simulink model "AnomalyResponseDelay"  (R2017b)
settings: Solver=FixedStepAuto  StartTime=0.0  StopTime=tfin  FixedStep=dT  MinStep=1e-5  RelTol=1e-6
values from neighbouring files (symbols this model uses):
  gamma = 10    [AnomalyResponseSim.m]
  tau = SP.tau    [AnomalyResponseSim.m]    (also in thesis_plots.m)
  ts = SP.ts    [AnomalyResponseSim.m]    (also in thesis_plots.m)
  ts_rm = SP.ts_rm    [AnomalyResponseSim.m]    (also in thesis_plots.m)
undefined symbols (not defined in the file or in its folder): Am, Am_3d, Ap, Bm, Bm_3d, Bp, dT, gamma_3d_q, gamma_3d_th, Lm, Lm_3d, P, P_3d, q0, q_0, Theta_0, theta_0_1, theta_0_2
libraries: vrlib x14, simulink x4
settings Model: Creator=ben  LastModifiedBy=ben
settings SolverCC: ShapePreserveControl=EnableAll  ZeroCrossControl=EnableAll
settings DataIOCC: SaveOutput=off  SignalLogging=off  DSMLogging=off  ReturnWorkspaceOutputs=on  ReturnWorkspaceOutputsName=simout
settings CodeAppCC: StateflowObjectComments=on

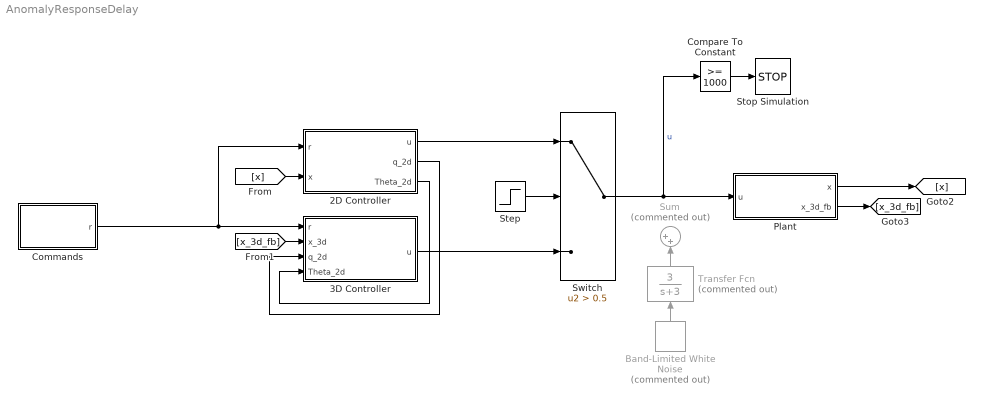
== system AnomalyResponseDelay ==
  2D Controller : Subsystem
  3D Controller : Subsystem
  Band-Limited White Noise : simulink/Sources/Band-Limited White Noise  Commented=on  Cov=[0.2]  Ts=0.05  seed=[23341]
  Commands : Subsystem
  Compare To Constant : simulink/Logic and Bit Operations/Compare To Constant  relop=>=  const=1000  OutDataTypeStr=boolean
  Plant : Subsystem
  Step : Step  Time=ts_rm  Before=1  After=0  SampleTime=0
  Stop Simulation : Stop
  Sum : Sum  Commented=on  Inputs=|++
  Switch : Switch  Criteria=u2 > Threshold  Threshold=0.5
  Transfer Fcn : TransferFcn  Commented=on  Numerator=[3]  Denominator=[1 3]
  wires:
  Plant/1(x) -> [x]
  Plant/2(x_3d_fb) -> [x_3d_fb]
  [x] -> 2D Controller/2(x)
  [x_3d_fb] -> 3D Controller/2(x_3d)
  Step/1 -> Switch/2
  Switch/1 -> Compare To Constant/1, Plant/1(u)  "u"
  3D Controller/1(u) -> Switch/3
  2D Controller/1(u) -> Switch/1
  2D Controller/3(Theta_2d) -> 3D Controller/4(Theta_2d)
  2D Controller/2(q_2d) -> 3D Controller/3(q_2d)
  Commands/1(r) -> 2D Controller/1(r), 3D Controller/1(r)
  Band-Limited White Noise/1 -> Transfer Fcn/1
  Transfer Fcn/1 -> Sum/2
  Compare To Constant/1 -> Stop Simulation/1

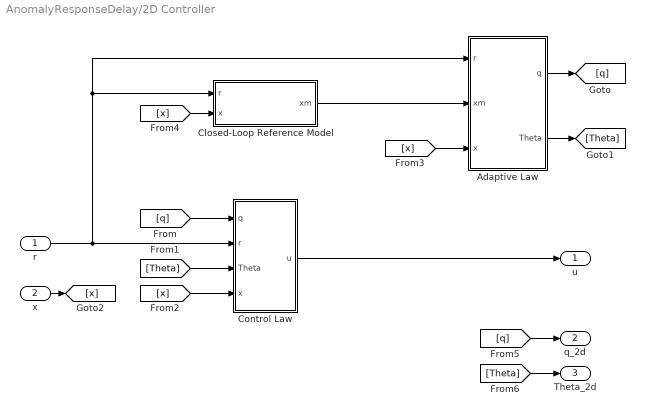
== system AnomalyResponseDelay/2D Controller ==
  r : Inport
  x : Inport  Port=2
  Adaptive Law : Subsystem
  Closed-Loop Reference Model : Subsystem
  Control Law : Subsystem
  u : Outport
  q_2d : Outport  Port=2
  Theta_2d : Outport  Port=3
  wires:
  Closed-Loop Reference Model/1(xm) -> Adaptive Law/2(xm)
  [x] -> Control Law/4(x)
  [q] -> Control Law/1(q)
  [Theta] -> Control Law/3(Theta)
  Adaptive Law/2(Theta) -> [Theta]
  r/1 -> Closed-Loop Reference Model/1(r), Adaptive Law/1(r), Control Law/2(r)
  [x] -> Closed-Loop Reference Model/2(x)
  [x] -> Adaptive Law/3(x)
  Adaptive Law/1(q) -> [q]
  Control Law/1(u) -> u/1
  x/1 -> [x]
  [q] -> q_2d/1
  [Theta] -> Theta_2d/1

== system AnomalyResponseDelay/3D Controller ==
  r : Inport
  x_3d : Inport  Port=2
  q_2d : Inport  Port=3
  Theta_2d : Inport  Port=4
  Adaptive Law : Subsystem
  Closed-Loop Reference Model : Subsystem
  Control Law : Subsystem
  u : Outport
  wires:
  Control Law/1(u) -> u/1
  Adaptive Law/1(q) -> [q_3d]
  [x_3d] -> Adaptive Law/3(x)
  [x_3d] -> Closed-Loop Reference Model/2(x)
  r/1 -> Control Law/2(r), Adaptive Law/1(r), Closed-Loop Reference Model/1(r)
  Adaptive Law/2(Theta) -> [Theta_3d]
  [Theta_3d] -> Control Law/3(Theta)
  [q_3d] -> Control Law/1(q)
  [x_3d] -> Control Law/4(x)
  Closed-Loop Reference Model/1(xm) -> Adaptive Law/2(xm)
  x_3d/1 -> [x_3d]
  Theta_2d/1 -> Adaptive Law/5(Theta_2d)
  q_2d/1 -> Adaptive Law/4(q_2d)

== system AnomalyResponseDelay/Commands ==
  From Workspace : FromWorkspace  VariableName=r_timed  SampleTime=0  Interpolate=off  OutputAfterFinalValue=Setting to zero
  To Workspace : ToWorkspace  VariableName=r  SampleTime=-1
      settings: Save2DSignal=2-D array (concatenate along first dimension)
  r : Outport
  wires:
  From Workspace/1 -> To Workspace/1, r/1

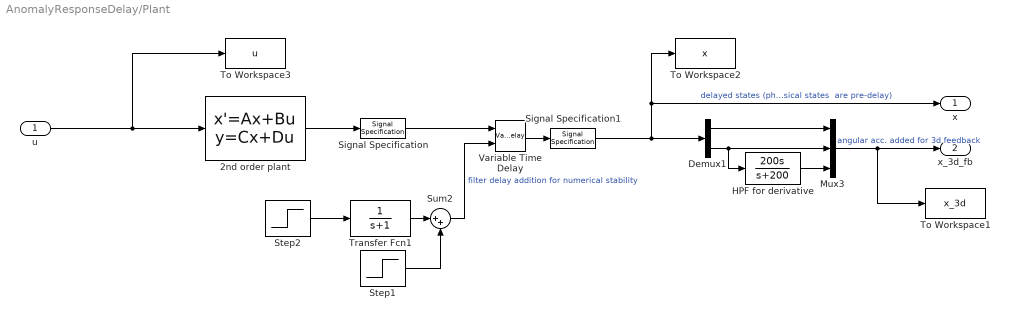
== system AnomalyResponseDelay/Plant ==
  u : Inport
  2nd order plant : StateSpace  A=Ap  B=Bp  C=eye(2)  D=[0; 0]  InitialCondition=0
  Demux1 : Demux  Outputs=[1 1]
  HPF for derivative : TransferFcn  Numerator=[200 0]  Denominator=[1 200]
  Mux3 : Mux  Inputs=[1 1 1]
  Signal Specification : SignalSpecification  Dimensions=[2 1]
  Signal Specification1 : SignalSpecification  Dimensions=[2 1]
  Step1 : Step  Time=ts  After=dT  SampleTime=0
  Step2 : Step  Time=ts  After=tau-dT  SampleTime=0
  Sum2 : Sum  Inputs=|++
  To Workspace1 : ToWorkspace  VariableName=x_3d  SampleTime=-1
      settings: Save2DSignal=2-D array (concatenate along first dimension)
  To Workspace2 : ToWorkspace  VariableName=x  SampleTime=-1
  To Workspace3 : ToWorkspace  VariableName=u  SampleTime=-1
      settings: Save2DSignal=2-D array (concatenate along first dimension)
  Transfer Fcn1 : TransferFcn  Denominator=[1 1]
  Variable Time Delay : VariableTransportDelay  MaximumDelay=tau*1.01  ZeroDelay=on
  x : Outport
  x_3d_fb : Outport  Port=2
  wires:
  Variable Time Delay/1 -> Signal Specification1/1
  Step2/1 -> Transfer Fcn1/1
  Sum2/1 -> Variable Time Delay/2  "filter delay addition for numerical stability"
  2nd order plant/1 -> Signal Specification/1
  u/1 -> 2nd order plant/1, To Workspace3/1
  Demux1/1 -> Mux3/1
  Demux1/2 -> HPF for derivative/1, Mux3/2
  HPF for derivative/1 -> Mux3/3
  Mux3/1 -> To Workspace1/1, x_3d_fb/1  "angular acc. added for 3d feedback"
  Signal Specification/1 -> Variable Time Delay/1
  Signal Specification1/1 -> Demux1/1, To Workspace2/1, x/1  "delayed states (physical states  are pre-delay)"
  Transfer Fcn1/1 -> Sum2/1
  Step1/1 -> Sum2/2

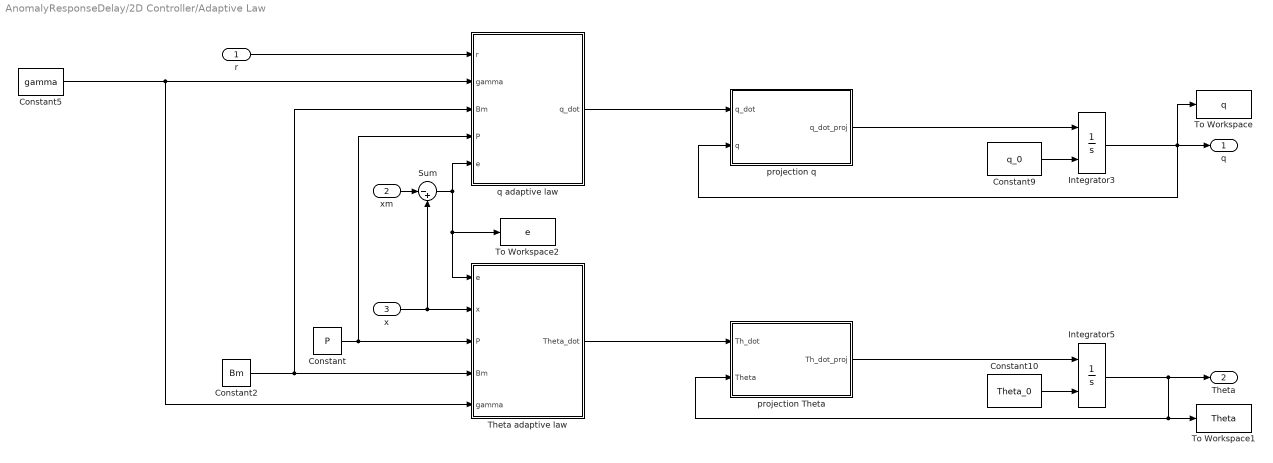
== system AnomalyResponseDelay/2D Controller/Adaptive Law ==
  r : Inport
  xm : Inport  Port=2  PortDimensions=[2,1]
  x : Inport  Port=3  PortDimensions=[2,1]
  Constant : Constant  Value=P  VectorParams1D=off
  Constant10 : Constant  Value=Theta_0  VectorParams1D=off
  Constant2 : Constant  Value=Bm  VectorParams1D=off
  Constant5 : Constant  Value=gamma  VectorParams1D=off
  Constant9 : Constant  Value=q_0  VectorParams1D=off
  Integrator3 : Integrator  InitialConditionSource=external  InitialCondition=q0
  Integrator5 : Integrator  InitialConditionSource=external
  Sum : Sum  Inputs=|-+
  Theta adaptive law : MATLAB Function  TreatAsAtomicUnit=on
  To Workspace : ToWorkspace  VariableName=q  SampleTime=-1
      settings: Save2DSignal=2-D array (concatenate along first dimension)
  To Workspace1 : ToWorkspace  VariableName=Theta  SampleTime=-1
      settings: Save2DSignal=2-D array (concatenate along first dimension)
  To Workspace2 : ToWorkspace  VariableName=e  SampleTime=-1
  projection Theta : Subsystem
  projection q : Subsystem
  q adaptive law : MATLAB Function  TreatAsAtomicUnit=on
  q : Outport
  Theta : Outport  Port=2
  wires:
  x/1 -> Theta adaptive law/2(x), Sum/2
  Constant/1 -> Theta adaptive law/3(P), q adaptive law/4(P)
  xm/1 -> Sum/1
  Sum/1 -> To Workspace2/1, Theta adaptive law/1(e), q adaptive law/5(e)
  Constant2/1 -> Theta adaptive law/4(Bm), q adaptive law/3(Bm)
  Constant5/1 -> Theta adaptive law/5(gamma), q adaptive law/2(gamma)
  r/1 -> q adaptive law/1(r)
  Constant9/1 -> Integrator3/2
  Integrator3/1 -> To Workspace/1, q/1, projection q/2(q)
  Constant10/1 -> Integrator5/2
  Integrator5/1 -> Theta/1, projection Theta/2(Theta), To Workspace1/1
  Theta adaptive law/1(Theta_dot) -> projection Theta/1(Th_dot)
  projection Theta/1(Th_dot_proj) -> Integrator5/1
  q adaptive law/1(q_dot) -> projection q/1(q_dot)
  projection q/1(q_dot_proj) -> Integrator3/1

== system AnomalyResponseDelay/2D Controller/Closed-Loop Reference Model ==
  r : Inport
  x : Inport  Port=2
  Am : Gain  Gain=Am  Multiplication=Matrix(K*u)
  Bm : Gain  Gain=Bm  Multiplication=Matrix(K*u)
  Integrator : Integrator
  Lm : Gain  Gain=Lm  Multiplication=Matrix(K*u)
  Sum2 : Sum  Inputs=-+|
  Sum3 : Sum  Inputs=-++
  To Workspace1 : ToWorkspace  VariableName=xm  SampleTime=-1
      settings: Save2DSignal=2-D array (concatenate along first dimension)
  xm : Outport
  wires:
  Integrator/1 -> Am/1, To Workspace1/1, xm/1, Sum2/1
  r/1 -> Bm/1
  x/1 -> Sum2/2
  Sum3/1 -> Integrator/1
  Bm/1 -> Sum3/2
  Lm/1 -> Sum3/1
  Sum2/1 -> Lm/1
  Am/1 -> Sum3/3

== system AnomalyResponseDelay/2D Controller/Control Law ==
  q : Inport
  r : Inport  Port=2
  Theta : Inport  Port=3
  x : Inport  Port=4
  Product : Product  Multiplication=Matrix(*)
  Sum : Sum  Inputs=|++
  q*r : Product
  u : Outport
  wires:
  x/1 -> Product/2
  q/1 -> q*r/1
  Product/1 -> Sum/2
  r/1 -> q*r/2
  q*r/1 -> Sum/1
  Sum/1 -> u/1
  Theta/1 -> Product/1

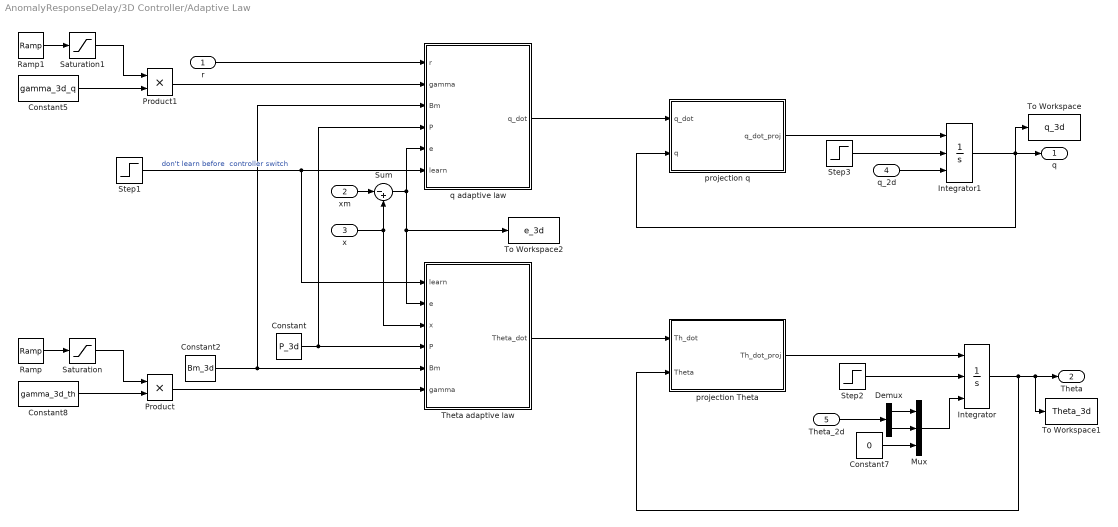
== system AnomalyResponseDelay/3D Controller/Adaptive Law ==
  r : Inport
  xm : Inport  Port=2  PortDimensions=[3,1]
  x : Inport  Port=3  PortDimensions=[3,1]
  q_2d : Inport  Port=4
  Theta_2d : Inport  Port=5
  Constant : Constant  Value=P_3d  VectorParams1D=off
  Constant2 : Constant  Value=Bm_3d  VectorParams1D=off
  Constant5 : Constant  Value=gamma_3d_q  VectorParams1D=off
  Constant7 : Constant  Value=0
  Constant8 : Constant  Value=gamma_3d_th  VectorParams1D=off
  Demux : Demux  Outputs=2
  Integrator : Integrator  ExternalReset=falling  InitialConditionSource=external
  Integrator1 : Integrator  ExternalReset=falling  InitialConditionSource=external  InitialCondition=q0
  Mux : Mux  Inputs=3
  Product : Product
  Product1 : Product
  Ramp : simulink/Sources/Ramp  slope=0.1  start=ts_rm  X0=0
  Ramp1 : simulink/Sources/Ramp  slope=0.1  start=ts_rm  X0=0
  Saturation : Saturate  UpperLimit=1  LowerLimit=0
  Saturation1 : Saturate  UpperLimit=1  LowerLimit=0
  Step1 : Step  Time=ts_rm  SampleTime=0
  Step2 : Step  Time=ts_rm  Before=0.5  After=-0.5  SampleTime=0
  Step3 : Step  Time=ts_rm  Before=0.5  After=-0.5  SampleTime=0
  Sum : Sum  Inputs=|-+
  Theta adaptive law : MATLAB Function  TreatAsAtomicUnit=on
  To Workspace : ToWorkspace  VariableName=q_3d  SampleTime=-1
      settings: Save2DSignal=2-D array (concatenate along first dimension)
  To Workspace1 : ToWorkspace  VariableName=Theta_3d  SampleTime=-1
      settings: Save2DSignal=2-D array (concatenate along first dimension)
  To Workspace2 : ToWorkspace  VariableName=e_3d  SampleTime=-1
  projection Theta : Subsystem
  projection q : Subsystem
  q adaptive law : MATLAB Function  TreatAsAtomicUnit=on
  q : Outport
  Theta : Outport  Port=2
  wires:
  r/1 -> q adaptive law/1(r)
  Constant2/1 -> q adaptive law/3(Bm), Theta adaptive law/5(Bm)
  Sum/1 -> q adaptive law/5(e), To Workspace2/1, Theta adaptive law/2(e)
  xm/1 -> Sum/1
  Constant/1 -> q adaptive law/4(P), Theta adaptive law/4(P)
  x/1 -> Theta adaptive law/3(x), Sum/2
  Step2/1 -> Integrator/2
  Step3/1 -> Integrator1/2
  Demux/1 -> Mux/1
  Demux/2 -> Mux/2
  Theta_2d/1 -> Demux/1
  Constant7/1 -> Mux/3
  Mux/1 -> Integrator/3
  Integrator1/1 -> projection q/2(q), q/1, To Workspace/1
  Integrator/1 -> projection Theta/2(Theta), Theta/1, To Workspace1/1
  q adaptive law/1(q_dot) -> projection q/1(q_dot)
  projection q/1(q_dot_proj) -> Integrator1/1
  Theta adaptive law/1(Theta_dot) -> projection Theta/1(Th_dot)
  projection Theta/1(Th_dot_proj) -> Integrator/1
  q_2d/1 -> Integrator1/3
  Product1/1 -> q adaptive law/2(gamma)
  Product/1 -> Theta adaptive law/6(gamma)
  Constant8/1 -> Product/2
  Ramp/1 -> Saturation/1
  Step1/1 -> Theta adaptive law/1(learn), q adaptive law/6(learn)  "don't learn before  controller switch"
  Saturation/1 -> Product/1
  Constant5/1 -> Product1/2
  Ramp1/1 -> Saturation1/1
  Saturation1/1 -> Product1/1

== system AnomalyResponseDelay/3D Controller/Closed-Loop Reference Model ==
  r : Inport
  x : Inport  Port=2
  Am : Gain  Gain=Am_3d  Multiplication=Matrix(K*u)
  Bm : Gain  Gain=Bm_3d  Multiplication=Matrix(K*u)
  Integrator : Integrator
  Lm : Gain  Gain=Lm_3d  Multiplication=Matrix(K*u)
  Sum2 : Sum  Inputs=-+|
  Sum3 : Sum  Inputs=-++
  To Workspace1 : ToWorkspace  VariableName=xm_3d  SampleTime=-1
      settings: Save2DSignal=2-D array (concatenate along first dimension)
  xm : Outport
  wires:
  Am/1 -> Sum3/3
  Sum2/1 -> Lm/1
  Lm/1 -> Sum3/1
  Bm/1 -> Sum3/2
  x/1 -> Sum2/2
  r/1 -> Bm/1
  Integrator/1 -> Sum2/1, xm/1, To Workspace1/1, Am/1
  Sum3/1 -> Integrator/1

== system AnomalyResponseDelay/3D Controller/Control Law ==
  q : Inport
  r : Inport  Port=2
  Theta : Inport  Port=3
  x : Inport  Port=4
  Product : Product  Multiplication=Matrix(*)
  Sum : Sum  Inputs=|++
  q*r : Product
  u : Outport
  wires:
  x/1 -> Product/2
  q/1 -> q*r/1
  Product/1 -> Sum/2
  r/1 -> q*r/2
  q*r/1 -> Sum/1
  Sum/1 -> u/1
  Theta/1 -> Product/1

== system AnomalyResponseDelay/2D Controller/Adaptive Law/projection Theta ==
  Th_dot : Inport
  Theta : Inport  Port=2
  Demux : Demux  Outputs=2
  Demux1 : Demux  Outputs=2
  Math Function : Math  Operator=transpose  SaturateOnIntegerOverflow=on
  Mux : Mux  Inputs=2
  Projection Block : Subsystem  mask{Epsilon=50, thetamax=200, Prcenter=0, Pr0=theta_0_1}
      mask prompts: thetamax "Bound (radius of the ball)"; Prcenter "Center of the Ball"; Pr0 "Initialization of integral"
      mask help:
      | Computes projection of the signal and safely integrate it.
      | Works both for scalar and vector signals.
      | It considers the parameter set as a ball at the specified location with
      | preset radius.
      mask init:
      | innerradius=thetamax/sqrt(1+Epsilon);
      | Intmax=thetamax+Prcenter;
      | Intmin=-thetamax+Prcenter;
      | Thetamax=innerradius;
  Projection Block1 : Subsystem  mask{Epsilon=100, thetamax=50, Prcenter=0, Pr0=theta_0_2}
      mask prompts: thetamax "Bound (radius of the ball)"; Prcenter "Center of the Ball"; Pr0 "Initialization of integral"
      mask help:
      | Computes projection of the signal and safely integrate it.
      | Works both for scalar and vector signals.
      | It considers the parameter set as a ball at the specified location with
      | preset radius.
      mask init:
      | innerradius=thetamax/sqrt(1+Epsilon);
      | Intmax=thetamax+Prcenter;
      | Intmin=-thetamax+Prcenter;
      | Thetamax=innerradius;
  Th_dot_proj : Outport
  wires:
  Math Function/1 -> Th_dot_proj/1
  Projection Block/1(proj) -> Mux/1
  Demux/1 -> Projection Block/2(y)
  Projection Block1/1(proj) -> Mux/2
  Demux/2 -> Projection Block1/2(y)
  Th_dot/1 -> Demux/1
  Mux/1 -> Math Function/1
  Theta/1 -> Demux1/1
  Demux1/1 -> Projection Block/1(theta)
  Demux1/2 -> Projection Block1/1(theta)

== system AnomalyResponseDelay/2D Controller/Adaptive Law/projection q ==
  q_dot : Inport
  q : Inport  Port=2
  Projection Block : Subsystem  mask{Epsilon=50, thetamax=200, Prcenter=0, Pr0=q_0}
      mask prompts: thetamax "Bound (radius of the ball)"; Prcenter "Center of the Ball"; Pr0 "Initialization of integral"
      mask help:
      | Computes projection of the signal and safely integrate it.
      | Works both for scalar and vector signals.
      | It considers the parameter set as a ball at the specified location with
      | preset radius.
      mask init:
      | innerradius=thetamax/sqrt(1+Epsilon);
      | Intmax=thetamax+Prcenter;
      | Intmin=-thetamax+Prcenter;
      | Thetamax=innerradius;
  q_dot_proj : Outport
  wires:
  q_dot/1 -> Projection Block/2(y)
  Projection Block/1(proj) -> q_dot_proj/1
  q/1 -> Projection Block/1(theta)

== system AnomalyResponseDelay/3D Controller/Adaptive Law/projection Theta ==
  Th_dot : Inport
  Theta : Inport  Port=2
  Demux : Demux  Outputs=3
  Demux1 : Demux  Outputs=3
  Math Function : Math  Operator=transpose  SaturateOnIntegerOverflow=on
  Mux : Mux  Inputs=3
  Projection Block : Subsystem  mask{Epsilon=50, thetamax=200, Prcenter=0, Pr0=theta_0_1}
      mask prompts: thetamax "Bound (radius of the ball)"; Prcenter "Center of the Ball"; Pr0 "Initialization of integral"
      mask help:
      | Computes projection of the signal and safely integrate it.
      | Works both for scalar and vector signals.
      | It considers the parameter set as a ball at the specified location with
      | preset radius.
      mask init:
      | innerradius=thetamax/sqrt(1+Epsilon);
      | Intmax=thetamax+Prcenter;
      | Intmin=-thetamax+Prcenter;
      | Thetamax=innerradius;
  Projection Block1 : Subsystem  mask{Epsilon=50, thetamax=75, Prcenter=0, Pr0=theta_0_2}
      mask prompts: thetamax "Bound (radius of the ball)"; Prcenter "Center of the Ball"; Pr0 "Initialization of integral"
      mask help:
      | Computes projection of the signal and safely integrate it.
      | Works both for scalar and vector signals.
      | It considers the parameter set as a ball at the specified location with
      | preset radius.
      mask init:
      | innerradius=thetamax/sqrt(1+Epsilon);
      | Intmax=thetamax+Prcenter;
      | Intmin=-thetamax+Prcenter;
      | Thetamax=innerradius;
  Projection Block2 : Subsystem  mask{Epsilon=5, thetamax=10, Prcenter=0, Pr0=0}
      mask prompts: thetamax "Bound (radius of the ball)"; Prcenter "Center of the Ball"; Pr0 "Initialization of integral"
      mask help:
      | Computes projection of the signal and safely integrate it.
      | Works both for scalar and vector signals.
      | It considers the parameter set as a ball at the specified location with
      | preset radius.
      mask init:
      | innerradius=thetamax/sqrt(1+Epsilon);
      | Intmax=thetamax+Prcenter;
      | Intmin=-thetamax+Prcenter;
      | Thetamax=innerradius;
  Th_dot_proj : Outport
  wires:
  Math Function/1 -> Th_dot_proj/1
  Projection Block/1(proj) -> Mux/1
  Demux/1 -> Projection Block/2(y)
  Projection Block1/1(proj) -> Mux/2
  Demux/2 -> Projection Block1/2(y)
  Th_dot/1 -> Demux/1
  Mux/1 -> Math Function/1
  Theta/1 -> Demux1/1
  Demux1/1 -> Projection Block/1(theta)
  Demux1/2 -> Projection Block1/1(theta)
  Projection Block2/1(proj) -> Mux/3
  Demux/3 -> Projection Block2/2(y)
  Demux1/3 -> Projection Block2/1(theta)

== system AnomalyResponseDelay/3D Controller/Adaptive Law/projection q ==
  q_dot : Inport
  q : Inport  Port=2
  Projection Block : Subsystem  mask{Epsilon=50, thetamax=200, Prcenter=0, Pr0=q_0}
      mask prompts: thetamax "Bound (radius of the ball)"; Prcenter "Center of the Ball"; Pr0 "Initialization of integral"
      mask help:
      | Computes projection of the signal and safely integrate it.
      | Works both for scalar and vector signals.
      | It considers the parameter set as a ball at the specified location with
      | preset radius.
      mask init:
      | innerradius=thetamax/sqrt(1+Epsilon);
      | Intmax=thetamax+Prcenter;
      | Intmin=-thetamax+Prcenter;
      | Thetamax=innerradius;
  q_dot_proj : Outport
  wires:
  q_dot/1 -> Projection Block/2(y)
  Projection Block/1(proj) -> q_dot_proj/1
  q/1 -> Projection Block/1(theta)

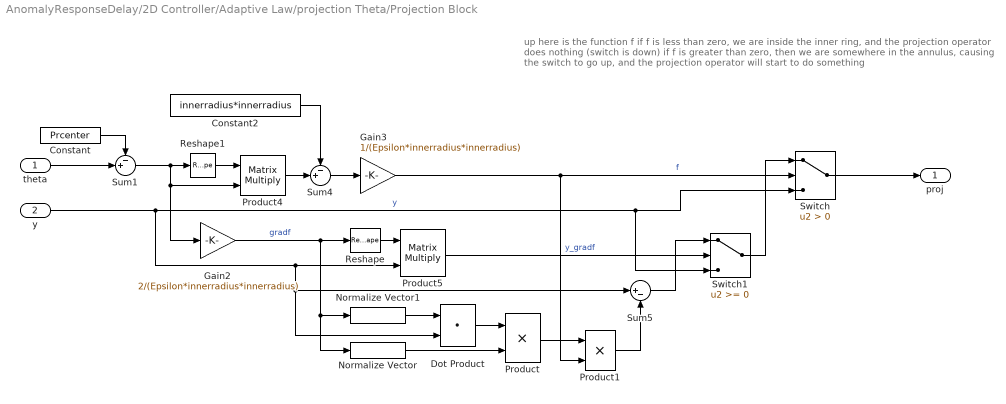
== system AnomalyResponseDelay/2D Controller/Adaptive Law/projection Theta/Projection Block ==
  note: up here is the function f
      | if f is less than zero, we are inside the inner ring, and the projection operator does nothing (switch is down)
      | if f is greater than zero, then we are somewhere in the annulus, causing the switch to go up, and the projection operator will start to do something
  theta : Inport
  y : Inport  Port=2
  Constant : Constant  Value=Prcenter
  Constant2 : Constant  Value=innerradius*innerradius
  Dot Product : DotProduct  InputSameDT=on  OutDataTypeStr=Inherit: Inherit via internal rule
  Gain2 : Gain  Gain=2/(Epsilon*innerradius*innerradius)
  Gain3 : Gain  Gain=1/(Epsilon*innerradius*innerradius)
  Normalize Vector : vrlib/Utilities/Normalize Vector  maxzero=0
      settings: SourceProductName=Simulink 3D Animation  SourceProductBaseCode=VR
  Normalize Vector1 : vrlib/Utilities/Normalize Vector  maxzero=0
      settings: SourceProductName=Simulink 3D Animation  SourceProductBaseCode=VR
  Product : Product  RndMeth=Zero
  Product1 : Product  RndMeth=Zero
  Product4 : Product  Multiplication=Matrix(*)  RndMeth=Zero
  Product5 : Product  Multiplication=Matrix(*)  RndMeth=Zero
  Reshape : Reshape  OutputDimensionality=Row vector (2-D)
  Reshape1 : Reshape  OutputDimensionality=Row vector (2-D)
  Sum1 : Sum  Inputs=-+|
  Sum4 : Sum  Inputs=-+|
  Sum5 : Sum  Inputs=|+-
  Switch : Switch  Criteria=u2 > Threshold
  Switch1 : Switch
  proj : Outport
  wires:
  Sum5/1 -> Switch1/1
  Sum4/1 -> Gain3/1
  Constant2/1 -> Sum4/1
  Product4/1 -> Sum4/2
  Constant/1 -> Sum1/1
  Sum1/1 -> Gain2/1, Product4/2, Reshape1/1
  theta/1 -> Sum1/2
  Product1/1 -> Sum5/2
  Product/1 -> Product1/1
  Normalize Vector/1 -> Product/2
  Dot Product/1 -> Product/1
  Normalize Vector1/1 -> Dot Product/1
  Reshape1/1 -> Product4/1
  Reshape/1 -> Product5/1
  Gain2/1 -> Normalize Vector/1, Normalize Vector1/1, Reshape/1  "gradf"
  Gain3/1 -> Product1/2, Switch/2  "f"
  Product5/1 -> Switch1/2  "y_gradf"
  Switch/1 -> proj/1
  y/1 -> Switch/3, Switch1/3, Dot Product/2, Sum5/1, Product5/2  "y"
  Switch1/1 -> Switch/1

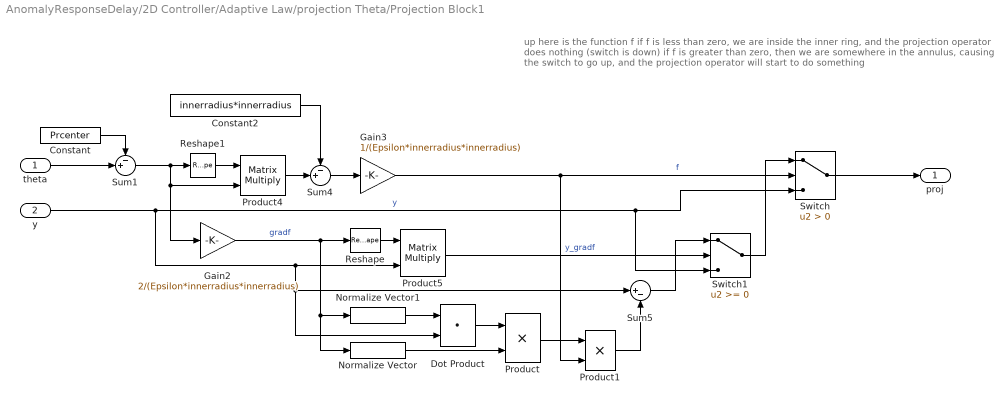
== system AnomalyResponseDelay/2D Controller/Adaptive Law/projection Theta/Projection Block1 ==
  note: up here is the function f
      | if f is less than zero, we are inside the inner ring, and the projection operator does nothing (switch is down)
      | if f is greater than zero, then we are somewhere in the annulus, causing the switch to go up, and the projection operator will start to do something
  theta : Inport
  y : Inport  Port=2
  Constant : Constant  Value=Prcenter
  Constant2 : Constant  Value=innerradius*innerradius
  Dot Product : DotProduct  InputSameDT=on  OutDataTypeStr=Inherit: Inherit via internal rule
  Gain2 : Gain  Gain=2/(Epsilon*innerradius*innerradius)
  Gain3 : Gain  Gain=1/(Epsilon*innerradius*innerradius)
  Normalize Vector : vrlib/Utilities/Normalize Vector  maxzero=0
      settings: SourceProductName=Simulink 3D Animation  SourceProductBaseCode=VR
  Normalize Vector1 : vrlib/Utilities/Normalize Vector  maxzero=0
      settings: SourceProductName=Simulink 3D Animation  SourceProductBaseCode=VR
  Product : Product  RndMeth=Zero
  Product1 : Product  RndMeth=Zero
  Product4 : Product  Multiplication=Matrix(*)  RndMeth=Zero
  Product5 : Product  Multiplication=Matrix(*)  RndMeth=Zero
  Reshape : Reshape  OutputDimensionality=Row vector (2-D)
  Reshape1 : Reshape  OutputDimensionality=Row vector (2-D)
  Sum1 : Sum  Inputs=-+|
  Sum4 : Sum  Inputs=-+|
  Sum5 : Sum  Inputs=|+-
  Switch : Switch  Criteria=u2 > Threshold
  Switch1 : Switch
  proj : Outport
  wires:
  Sum5/1 -> Switch1/1
  Sum4/1 -> Gain3/1
  Constant2/1 -> Sum4/1
  Product4/1 -> Sum4/2
  Constant/1 -> Sum1/1
  Sum1/1 -> Gain2/1, Product4/2, Reshape1/1
  theta/1 -> Sum1/2
  Product1/1 -> Sum5/2
  Product/1 -> Product1/1
  Normalize Vector/1 -> Product/2
  Dot Product/1 -> Product/1
  Normalize Vector1/1 -> Dot Product/1
  Reshape1/1 -> Product4/1
  Reshape/1 -> Product5/1
  Gain2/1 -> Normalize Vector/1, Normalize Vector1/1, Reshape/1  "gradf"
  Gain3/1 -> Product1/2, Switch/2  "f"
  Product5/1 -> Switch1/2  "y_gradf"
  Switch/1 -> proj/1
  y/1 -> Switch/3, Switch1/3, Dot Product/2, Sum5/1, Product5/2  "y"
  Switch1/1 -> Switch/1

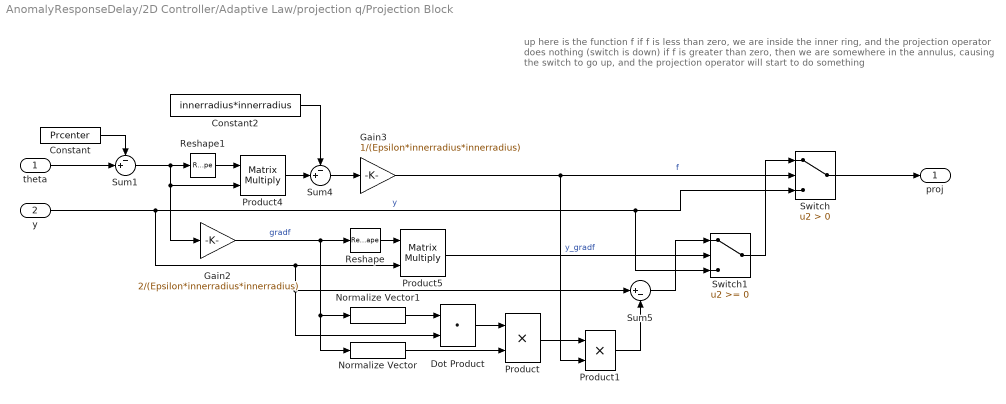
== system AnomalyResponseDelay/2D Controller/Adaptive Law/projection q/Projection Block ==
  note: up here is the function f
      | if f is less than zero, we are inside the inner ring, and the projection operator does nothing (switch is down)
      | if f is greater than zero, then we are somewhere in the annulus, causing the switch to go up, and the projection operator will start to do something
  theta : Inport
  y : Inport  Port=2
  Constant : Constant  Value=Prcenter
  Constant2 : Constant  Value=innerradius*innerradius
  Dot Product : DotProduct  InputSameDT=on  OutDataTypeStr=Inherit: Inherit via internal rule
  Gain2 : Gain  Gain=2/(Epsilon*innerradius*innerradius)
  Gain3 : Gain  Gain=1/(Epsilon*innerradius*innerradius)
  Normalize Vector : vrlib/Utilities/Normalize Vector  maxzero=0
      settings: SourceProductName=Simulink 3D Animation  SourceProductBaseCode=VR
  Normalize Vector1 : vrlib/Utilities/Normalize Vector  maxzero=0
      settings: SourceProductName=Simulink 3D Animation  SourceProductBaseCode=VR
  Product : Product  RndMeth=Zero
  Product1 : Product  RndMeth=Zero
  Product4 : Product  Multiplication=Matrix(*)  RndMeth=Zero
  Product5 : Product  Multiplication=Matrix(*)  RndMeth=Zero
  Reshape : Reshape  OutputDimensionality=Row vector (2-D)
  Reshape1 : Reshape  OutputDimensionality=Row vector (2-D)
  Sum1 : Sum  Inputs=-+|
  Sum4 : Sum  Inputs=-+|
  Sum5 : Sum  Inputs=|+-
  Switch : Switch  Criteria=u2 > Threshold
  Switch1 : Switch
  proj : Outport
  wires:
  Sum5/1 -> Switch1/1
  Sum4/1 -> Gain3/1
  Constant2/1 -> Sum4/1
  Product4/1 -> Sum4/2
  Constant/1 -> Sum1/1
  Sum1/1 -> Gain2/1, Product4/2, Reshape1/1
  theta/1 -> Sum1/2
  Product1/1 -> Sum5/2
  Product/1 -> Product1/1
  Normalize Vector/1 -> Product/2
  Dot Product/1 -> Product/1
  Normalize Vector1/1 -> Dot Product/1
  Reshape1/1 -> Product4/1
  Reshape/1 -> Product5/1
  Gain2/1 -> Normalize Vector/1, Normalize Vector1/1, Reshape/1  "gradf"
  Gain3/1 -> Product1/2, Switch/2  "f"
  Product5/1 -> Switch1/2  "y_gradf"
  Switch/1 -> proj/1
  y/1 -> Switch/3, Switch1/3, Dot Product/2, Sum5/1, Product5/2  "y"
  Switch1/1 -> Switch/1

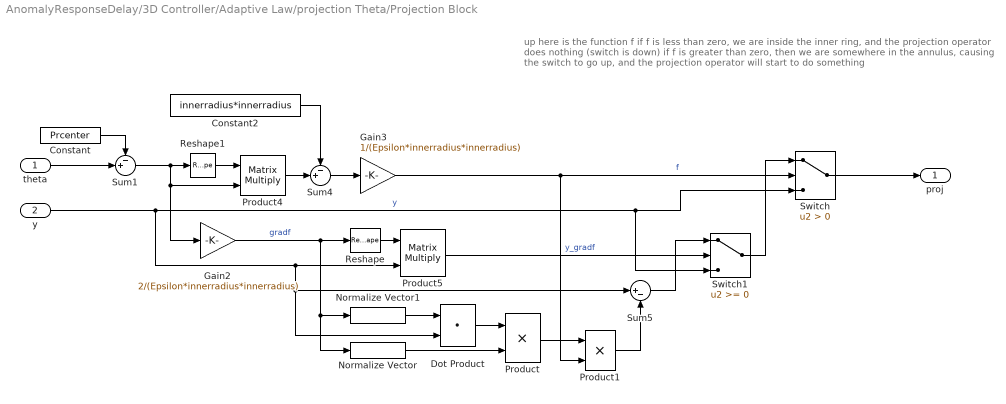
== system AnomalyResponseDelay/3D Controller/Adaptive Law/projection Theta/Projection Block ==
  note: up here is the function f
      | if f is less than zero, we are inside the inner ring, and the projection operator does nothing (switch is down)
      | if f is greater than zero, then we are somewhere in the annulus, causing the switch to go up, and the projection operator will start to do something
  theta : Inport
  y : Inport  Port=2
  Constant : Constant  Value=Prcenter
  Constant2 : Constant  Value=innerradius*innerradius
  Dot Product : DotProduct  InputSameDT=on  OutDataTypeStr=Inherit: Inherit via internal rule
  Gain2 : Gain  Gain=2/(Epsilon*innerradius*innerradius)
  Gain3 : Gain  Gain=1/(Epsilon*innerradius*innerradius)
  Normalize Vector : vrlib/Utilities/Normalize Vector  maxzero=0
      settings: SourceProductName=Simulink 3D Animation  SourceProductBaseCode=VR
  Normalize Vector1 : vrlib/Utilities/Normalize Vector  maxzero=0
      settings: SourceProductName=Simulink 3D Animation  SourceProductBaseCode=VR
  Product : Product  RndMeth=Zero
  Product1 : Product  RndMeth=Zero
  Product4 : Product  Multiplication=Matrix(*)  RndMeth=Zero
  Product5 : Product  Multiplication=Matrix(*)  RndMeth=Zero
  Reshape : Reshape  OutputDimensionality=Row vector (2-D)
  Reshape1 : Reshape  OutputDimensionality=Row vector (2-D)
  Sum1 : Sum  Inputs=-+|
  Sum4 : Sum  Inputs=-+|
  Sum5 : Sum  Inputs=|+-
  Switch : Switch  Criteria=u2 > Threshold
  Switch1 : Switch
  proj : Outport
  wires:
  Sum5/1 -> Switch1/1
  Sum4/1 -> Gain3/1
  Constant2/1 -> Sum4/1
  Product4/1 -> Sum4/2
  Constant/1 -> Sum1/1
  Sum1/1 -> Gain2/1, Product4/2, Reshape1/1
  theta/1 -> Sum1/2
  Product1/1 -> Sum5/2
  Product/1 -> Product1/1
  Normalize Vector/1 -> Product/2
  Dot Product/1 -> Product/1
  Normalize Vector1/1 -> Dot Product/1
  Reshape1/1 -> Product4/1
  Reshape/1 -> Product5/1
  Gain2/1 -> Normalize Vector/1, Normalize Vector1/1, Reshape/1  "gradf"
  Gain3/1 -> Product1/2, Switch/2  "f"
  Product5/1 -> Switch1/2  "y_gradf"
  Switch/1 -> proj/1
  y/1 -> Switch/3, Switch1/3, Dot Product/2, Sum5/1, Product5/2  "y"
  Switch1/1 -> Switch/1

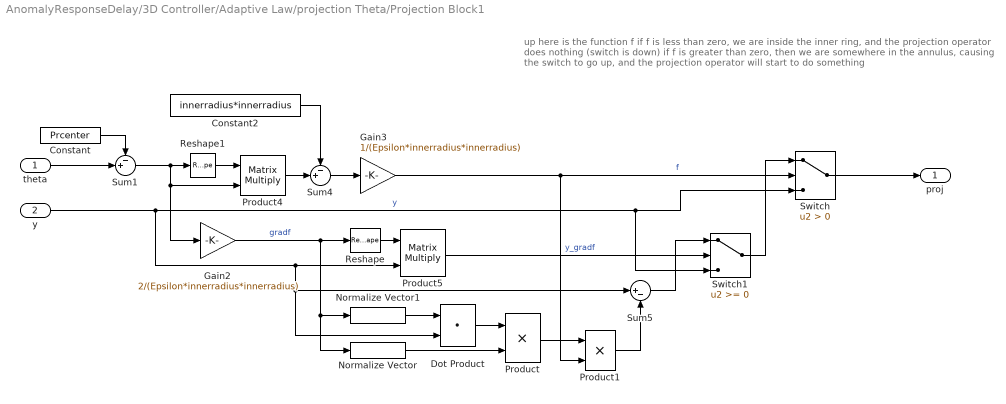
== system AnomalyResponseDelay/3D Controller/Adaptive Law/projection Theta/Projection Block1 ==
  note: up here is the function f
      | if f is less than zero, we are inside the inner ring, and the projection operator does nothing (switch is down)
      | if f is greater than zero, then we are somewhere in the annulus, causing the switch to go up, and the projection operator will start to do something
  theta : Inport
  y : Inport  Port=2
  Constant : Constant  Value=Prcenter
  Constant2 : Constant  Value=innerradius*innerradius
  Dot Product : DotProduct  InputSameDT=on  OutDataTypeStr=Inherit: Inherit via internal rule
  Gain2 : Gain  Gain=2/(Epsilon*innerradius*innerradius)
  Gain3 : Gain  Gain=1/(Epsilon*innerradius*innerradius)
  Normalize Vector : vrlib/Utilities/Normalize Vector  maxzero=0
      settings: SourceProductName=Simulink 3D Animation  SourceProductBaseCode=VR
  Normalize Vector1 : vrlib/Utilities/Normalize Vector  maxzero=0
      settings: SourceProductName=Simulink 3D Animation  SourceProductBaseCode=VR
  Product : Product  RndMeth=Zero
  Product1 : Product  RndMeth=Zero
  Product4 : Product  Multiplication=Matrix(*)  RndMeth=Zero
  Product5 : Product  Multiplication=Matrix(*)  RndMeth=Zero
  Reshape : Reshape  OutputDimensionality=Row vector (2-D)
  Reshape1 : Reshape  OutputDimensionality=Row vector (2-D)
  Sum1 : Sum  Inputs=-+|
  Sum4 : Sum  Inputs=-+|
  Sum5 : Sum  Inputs=|+-
  Switch : Switch  Criteria=u2 > Threshold
  Switch1 : Switch
  proj : Outport
  wires:
  Sum5/1 -> Switch1/1
  Sum4/1 -> Gain3/1
  Constant2/1 -> Sum4/1
  Product4/1 -> Sum4/2
  Constant/1 -> Sum1/1
  Sum1/1 -> Gain2/1, Product4/2, Reshape1/1
  theta/1 -> Sum1/2
  Product1/1 -> Sum5/2
  Product/1 -> Product1/1
  Normalize Vector/1 -> Product/2
  Dot Product/1 -> Product/1
  Normalize Vector1/1 -> Dot Product/1
  Reshape1/1 -> Product4/1
  Reshape/1 -> Product5/1
  Gain2/1 -> Normalize Vector/1, Normalize Vector1/1, Reshape/1  "gradf"
  Gain3/1 -> Product1/2, Switch/2  "f"
  Product5/1 -> Switch1/2  "y_gradf"
  Switch/1 -> proj/1
  y/1 -> Switch/3, Switch1/3, Dot Product/2, Sum5/1, Product5/2  "y"
  Switch1/1 -> Switch/1

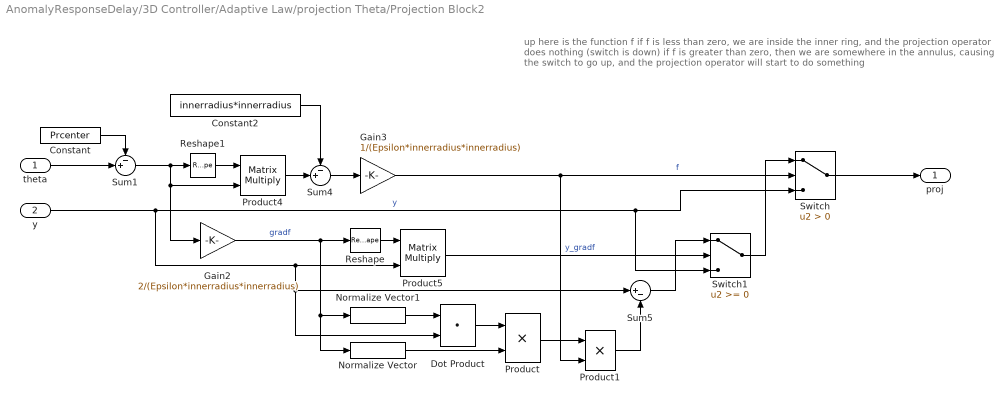
== system AnomalyResponseDelay/3D Controller/Adaptive Law/projection Theta/Projection Block2 ==
  note: up here is the function f
      | if f is less than zero, we are inside the inner ring, and the projection operator does nothing (switch is down)
      | if f is greater than zero, then we are somewhere in the annulus, causing the switch to go up, and the projection operator will start to do something
  theta : Inport
  y : Inport  Port=2
  Constant : Constant  Value=Prcenter
  Constant2 : Constant  Value=innerradius*innerradius
  Dot Product : DotProduct  InputSameDT=on  OutDataTypeStr=Inherit: Inherit via internal rule
  Gain2 : Gain  Gain=2/(Epsilon*innerradius*innerradius)
  Gain3 : Gain  Gain=1/(Epsilon*innerradius*innerradius)
  Normalize Vector : vrlib/Utilities/Normalize Vector  maxzero=0
      settings: SourceProductName=Simulink 3D Animation  SourceProductBaseCode=VR
  Normalize Vector1 : vrlib/Utilities/Normalize Vector  maxzero=0
      settings: SourceProductName=Simulink 3D Animation  SourceProductBaseCode=VR
  Product : Product  RndMeth=Zero
  Product1 : Product  RndMeth=Zero
  Product4 : Product  Multiplication=Matrix(*)  RndMeth=Zero
  Product5 : Product  Multiplication=Matrix(*)  RndMeth=Zero
  Reshape : Reshape  OutputDimensionality=Row vector (2-D)
  Reshape1 : Reshape  OutputDimensionality=Row vector (2-D)
  Sum1 : Sum  Inputs=-+|
  Sum4 : Sum  Inputs=-+|
  Sum5 : Sum  Inputs=|+-
  Switch : Switch  Criteria=u2 > Threshold
  Switch1 : Switch
  proj : Outport
  wires:
  Sum5/1 -> Switch1/1
  Sum4/1 -> Gain3/1
  Constant2/1 -> Sum4/1
  Product4/1 -> Sum4/2
  Constant/1 -> Sum1/1
  Sum1/1 -> Gain2/1, Product4/2, Reshape1/1
  theta/1 -> Sum1/2
  Product1/1 -> Sum5/2
  Product/1 -> Product1/1
  Normalize Vector/1 -> Product/2
  Dot Product/1 -> Product/1
  Normalize Vector1/1 -> Dot Product/1
  Reshape1/1 -> Product4/1
  Reshape/1 -> Product5/1
  Gain2/1 -> Normalize Vector/1, Normalize Vector1/1, Reshape/1  "gradf"
  Gain3/1 -> Product1/2, Switch/2  "f"
  Product5/1 -> Switch1/2  "y_gradf"
  Switch/1 -> proj/1
  y/1 -> Switch/3, Switch1/3, Dot Product/2, Sum5/1, Product5/2  "y"
  Switch1/1 -> Switch/1

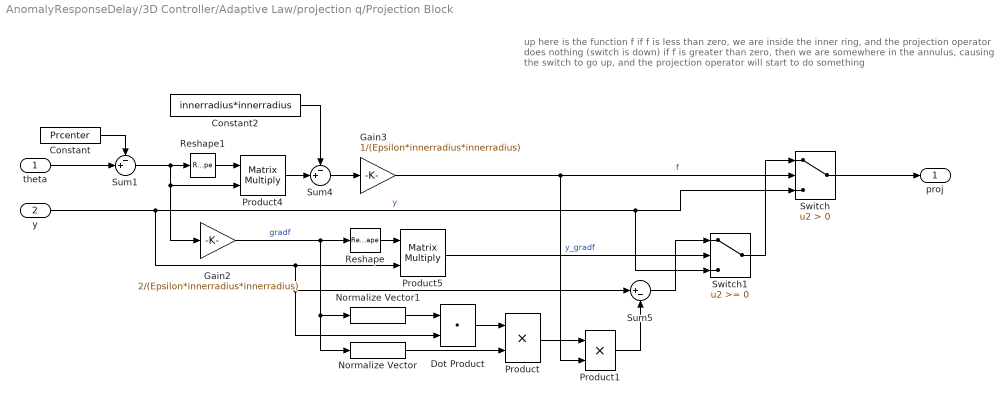
== system AnomalyResponseDelay/3D Controller/Adaptive Law/projection q/Projection Block ==
  note: up here is the function f
      | if f is less than zero, we are inside the inner ring, and the projection operator does nothing (switch is down)
      | if f is greater than zero, then we are somewhere in the annulus, causing the switch to go up, and the projection operator will start to do something
  theta : Inport
  y : Inport  Port=2
  Constant : Constant  Value=Prcenter
  Constant2 : Constant  Value=innerradius*innerradius
  Dot Product : DotProduct  InputSameDT=on  OutDataTypeStr=Inherit: Inherit via internal rule
  Gain2 : Gain  Gain=2/(Epsilon*innerradius*innerradius)
  Gain3 : Gain  Gain=1/(Epsilon*innerradius*innerradius)
  Normalize Vector : vrlib/Utilities/Normalize Vector  maxzero=0
      settings: SourceProductName=Simulink 3D Animation  SourceProductBaseCode=VR
  Normalize Vector1 : vrlib/Utilities/Normalize Vector  maxzero=0
      settings: SourceProductName=Simulink 3D Animation  SourceProductBaseCode=VR
  Product : Product  RndMeth=Zero
  Product1 : Product  RndMeth=Zero
  Product4 : Product  Multiplication=Matrix(*)  RndMeth=Zero
  Product5 : Product  Multiplication=Matrix(*)  RndMeth=Zero
  Reshape : Reshape  OutputDimensionality=Row vector (2-D)
  Reshape1 : Reshape  OutputDimensionality=Row vector (2-D)
  Sum1 : Sum  Inputs=-+|
  Sum4 : Sum  Inputs=-+|
  Sum5 : Sum  Inputs=|+-
  Switch : Switch  Criteria=u2 > Threshold
  Switch1 : Switch
  proj : Outport
  wires:
  Sum5/1 -> Switch1/1
  Sum4/1 -> Gain3/1
  Constant2/1 -> Sum4/1
  Product4/1 -> Sum4/2
  Constant/1 -> Sum1/1
  Sum1/1 -> Gain2/1, Product4/2, Reshape1/1
  theta/1 -> Sum1/2
  Product1/1 -> Sum5/2
  Product/1 -> Product1/1
  Normalize Vector/1 -> Product/2
  Dot Product/1 -> Product/1
  Normalize Vector1/1 -> Dot Product/1
  Reshape1/1 -> Product4/1
  Reshape/1 -> Product5/1
  Gain2/1 -> Normalize Vector/1, Normalize Vector1/1, Reshape/1  "gradf"
  Gain3/1 -> Product1/2, Switch/2  "f"
  Product5/1 -> Switch1/2  "y_gradf"
  Switch/1 -> proj/1
  y/1 -> Switch/3, Switch1/3, Dot Product/2, Sum5/1, Product5/2  "y"
  Switch1/1 -> Switch/1

== matlab function AnomalyResponseDelay/2D Controller/Adaptive Law/q adaptive law ==
  data: r input; gamma input; Bm input; P input; q_dot output; e input
function q_dot = fcn(r,gamma,Bm,P,e)
q_dot = - gamma * Bm' * P * e * r;

== matlab function AnomalyResponseDelay/2D Controller/Adaptive Law/Theta adaptive law ==
  data: e input; Theta_dot output; x input; P input; Bm input; gamma input
function Theta_dot = fcn(e,x,P,Bm,gamma)
Theta_dot = - gamma * Bm' * P * e * x';

== matlab function AnomalyResponseDelay/3D Controller/Adaptive Law/Theta adaptive law ==
  data: learn input; e input; Theta_dot output; x input; P input; Bm input; gamma input
function Theta_dot = fcn(learn,e,x,P,Bm,gamma)
% Theta_dot = - gamma * Bm' * P * e * x';
if learn == 1
    Theta_dot = - Bm' * gamma * P * e * x';
else
    Theta_dot = 0 * x';
end

== matlab function AnomalyResponseDelay/3D Controller/Adaptive Law/q adaptive law ==
  data: r input; gamma input; Bm input; P input; q_dot output; e input; learn input
function q_dot = fcn(r,gamma,Bm,P,e,learn)
if learn == 1
    q_dot = - gamma * Bm' * P * e * r;
else
    q_dot = 0;
end
